simulink model "History1NoActions"  (Simulink 9.0)
settings: Solver=ode45  StartTime=0.0  StopTime=10.0  RelTol=1e-3  EnableMultiTasking=on
settings Model: SuppressorTable=22 serialization::archive 11 0 6 0 0 0 0 0  Creator=scaife  LastModifiedBy=ktrinh  ExtModeAutoUpdateStatusClock=off
settings DataIOCC: LimitDataPoints=on  SignalLoggingSaveFormat=ModelDataLogs  SignalLoggingName=sigsOut
settings DebuggingCC: SaveWithParameterizedLinksMsg=none  SignalResolutionControl=TryResolveAllWithWarning  MultiTaskDSMMsg=warning  MultiTaskCondExecSysMsg=none  SFUnexpectedBacktrackingDiag=error  SFNoUnconditionalDefaultTransitionDiag=error
settings HardwareCC: TargetUnknown=on
settings SFSimCC: SimParseCustomCode=off
settings GRTTargetCC: CombineOutputUpdateFcns=off  GRTInterface=on

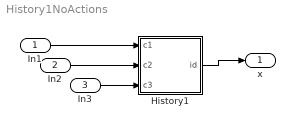
== system History1NoActions ==
  In1 : Inport  OutDataTypeStr=boolean
  In2 : Inport  Port=2  OutDataTypeStr=boolean
  In3 : Inport  Port=3  OutDataTypeStr=boolean
  History1 : Stateflow chart  TreatAsAtomicUnit=on
  x : Outport
  wires:
  History1/1(id) -> x/1
  In1/1 -> History1/1(c1)
  In3/1 -> History1/3(c3)
  In2/1 -> History1/2(c2)

== stateflow chart History1 ==
  state A
    (history)
    state A1/
      en: id=1;
    state A2/
      en: id=2;
    (default) -> A1
    A2 -> A1 : [c3]
    A1 -> A2 : [c3]
  state B
    (history)
    state B1/
      en: id=3;
    state B2/
      en: id=4;
    (default) -> B1
    B2 -> B1 : [c3]
    B1 -> B2 : [c3]
  (default) -> A
  A -> B : [c1]
  B -> A : [c2]
  data: c1 input boolean; c2 input boolean; c3 input boolean; id output double
